simulink model "mouter"  (R2022a)
settings: Solver=VariableStepAuto  StartTime=0.0  StopTime=10  RelTol=1e-3
values from neighbouring files (symbols this model uses):
  Ce = 0.556    [Untitled.m]    (also in liner.m)
  Ki = 5    [Untitled.m]    (also in liner.m = 1)
  Kn = 7.84    [Untitled.m]    (also in liner.m = 29.75)
  R = 0.6    [Untitled.m]    (also in liner.m)
  ti = 0.167    [Untitled.m]    (also in liner.m = 0.47)
  Tl = 0.167    [Untitled.m]    (also in liner.m)
  Tm = 0.282    [Untitled.m]    (also in liner.m)
  tn = 0.1    [Untitled.m]    (also in liner.m = 200)
  Ts = 0.01    [Untitled.m]    (also in liner.m)
settings Model: Creator=xinyu  LastModifiedBy=houtonglei
settings DebuggingCC: UnconnectedInputMsg=warning  UnconnectedOutputMsg=warning  UnconnectedLineMsg=warning
settings RTWCC: DLArmComputeVersion=19.05

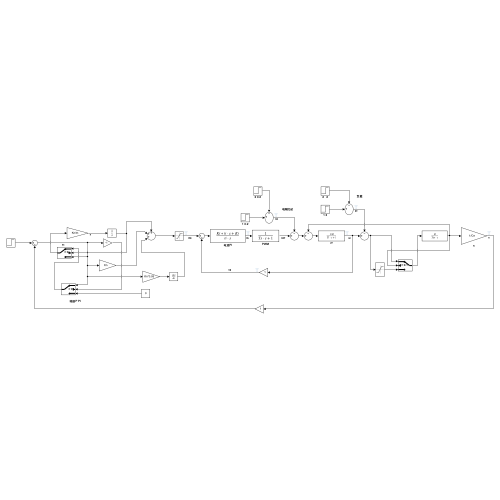
[thumbnail: Simulink's stored preview of the top-level diagram]
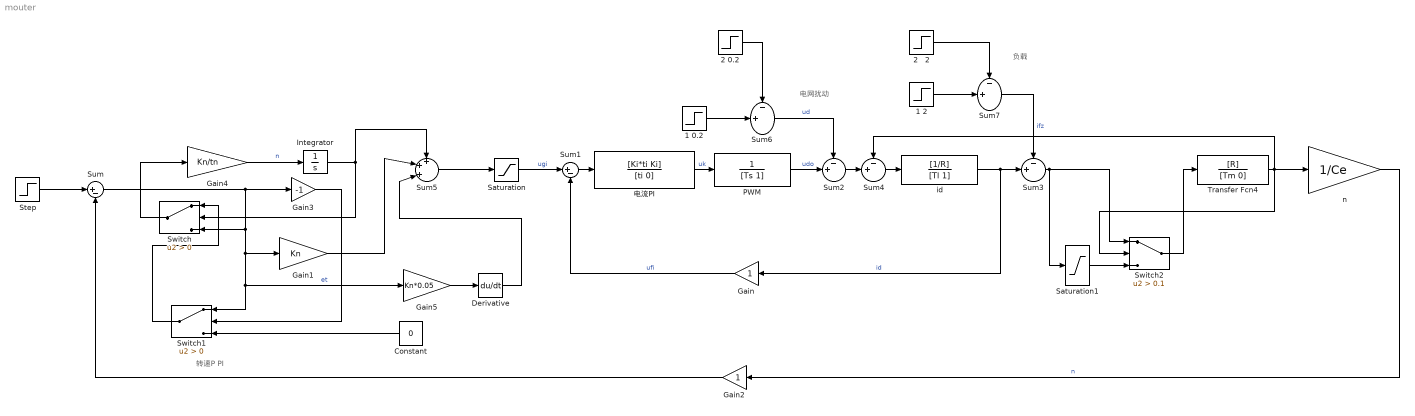
== system mouter ==
  note: 负载
  note: 转速P PI
  note: 电网扰动
  " 电流PI" : TransferFcn  Numerator=[Ki*ti Ki]  Denominator=[ti 0]  ContinuousStateAttributes='acr'
  1 0.2 : Step  After=0.2  SampleTime=0
  1 2 : Step  After=2  SampleTime=0
  2   2 : Step  Time=2  After=2  SampleTime=0
  2 0.2 : Step  Time=2  After=0.2  SampleTime=0
  Constant : Constant  Value=0
  Derivative : Derivative
  Gain : Gain
  Gain1 : Gain  Gain=Kn
  Gain2 : Gain
  Gain3 : Gain  Gain=-1
  Gain4 : Gain  Gain=Kn/tn
  Gain5 : Gain  Gain=Kn*0.05
  Integrator : Integrator
  PWM : TransferFcn  Denominator=[Ts 1]  ContinuousStateAttributes='pwm'
  Saturation : Saturate  UpperLimit=2.4  LowerLimit=-2.4
  Saturation1 : Saturate  UpperLimit=5  LowerLimit=0
  Step : Step  Time=0  After=2  SampleTime=0
  Sum : Sum  Inputs=|+-
  Sum1 : Sum  Inputs=|+-
  Sum{2..4,6..7} (5 alike) : Sum  Inputs=-+|
  Sum5 : Sum  Inputs=+++|
  Switch : Switch  Criteria=u2 > Threshold  SaturateOnIntegerOverflow=off  InputSameDT=off
  Switch1 : Switch  Criteria=u2 > Threshold  SaturateOnIntegerOverflow=off  InputSameDT=off
  Switch2 : Switch  Criteria=u2 > Threshold  Threshold=0.1  SaturateOnIntegerOverflow=off  InputSameDT=off
  Transfer Fcn4 : TransferFcn  Numerator=[R]  Denominator=[Tm 0]  ContinuousStateAttributes='inter'
  id : TransferFcn  Numerator=[1/R]  Denominator=[Tl 1]  ContinuousStateAttributes='mouter'
  n : Gain  Gain=1/Ce
  wires:
  2   2/1 -> Sum7/1
  Sum5/1 -> Saturation/1
  Sum/1 -> Gain3/1, Switch/3, Gain1/1, Gain5/1, Switch1/1  "et"
  Saturation1/1 -> Switch2/3
  1 0.2/1 -> Sum6/2
  2 0.2/1 -> Sum6/1
  " 电流PI"/1 -> PWM/1  "uk"
  Constant/1 -> Switch1/3
  PWM/1 -> Sum2/2  "udo"
  Saturation/1 -> Sum1/1  "ugi"
  id/1 -> Sum3/2, Gain/1  "id"
  Sum3/1 -> Switch2/1, Saturation1/1
  Sum1/1 -> " 电流PI"/1
  Gain4/1 -> Integrator/1  "n"
  Gain1/1 -> Sum5/2
  Gain3/1 -> Switch1/2
  1 2/1 -> Sum7/2
  Switch/1 -> Gain4/1
  Switch2/1 -> Transfer Fcn4/1
  Transfer Fcn4/1 -> Switch2/2, Sum4/1, n/1
  Sum4/1 -> id/1
  Switch1/1 -> Switch/1
  Gain/1 -> Sum1/2  "ufi"
  Sum2/1 -> Sum4/2
  Integrator/1 -> Switch/2, Sum5/1
  Step/1 -> Sum/1
  Gain2/1 -> Sum/2
  n/1 -> Gain2/1  "n"
  Gain5/1 -> Derivative/1
  Derivative/1 -> Sum5/3
  Sum6/1 -> Sum2/1  "ud"
  Sum7/1 -> Sum3/1  "ifz"
